simulink model "ControlerModel"  (R2022a)
settings: Solver=VariableStepAuto  StartTime=0.0  StopTime=4  RelTol=1e-3
libraries: simulink_extras x3
settings Model: Creator=Abdullah Syed  LastModifiedBy=Abdullah Syed

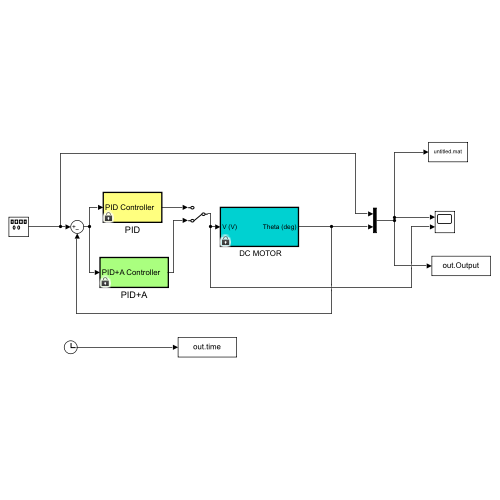
[thumbnail: Simulink's stored preview of the top-level diagram]
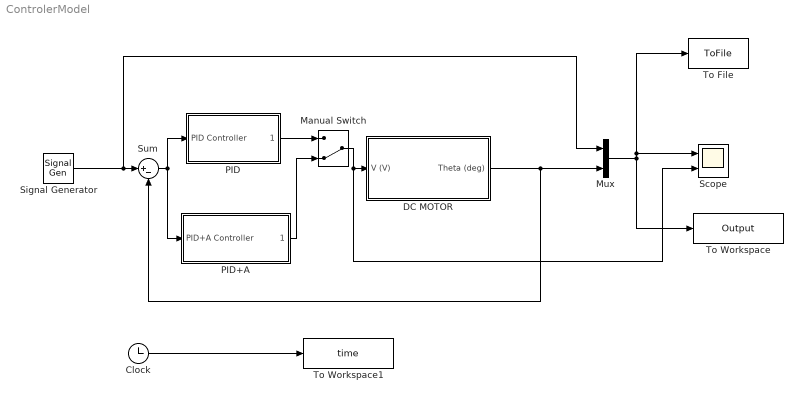
== system ControlerModel ==
  " DC MOTOR" : Subsystem  TreatAsAtomicUnit=on  mask(Single-Tank Nonlinear Model){La=2e-04, Ra=3.5, Jm=3.4700e-07, Bm=1.3319e-07}
      mask prompts: La "Armature Inductance - La (H)"; Ra "Armature Resistance - Ra (ohm)"; Jm "Motor Inertia - Jm (oz.in.sec^2)"; Bm "Motor Viscous Friction - Bm (N.m.sec)"
      mask help: The DC Motor model with saturaton and dead-zone nonlinearities.
      settings: MinAlgLoopOccurrences=on
  Clock : Clock
  Manual Switch : ManualSwitch  CurrentSetting=0
  Mux : Mux  Inputs=2
  PID : Subsystem  TreatAsAtomicUnit=on  mask{Kp=0.52, Ti=5, Td=0}
      mask prompts: Kp "Proportional Gain (Kp)"; Ti "Integral Time Constant (Ti)"; Td "Derivative Time Constant (Td)"
      mask help: This block implements continous PID controller in ideal structure.
      settings: MinAlgLoopOccurrences=on
  PID+A : Subsystem  TreatAsAtomicUnit=on  mask{Kp=0.45, Ti=1.5, Td=0, Kw=7}
      mask prompts: Kp "Proportional Gain (Kp)"; Ti "Integral Time Constant (Ti)"; Td "Derivative Time Constant (Td)"; Kw "Anti-Windup Gain (Kw)"
      mask help: This block implements continous PID controller in ideal structure.
      settings: MinAlgLoopOccurrences=on
  Scope : Scope  NumInputPorts=2
  Signal Generator : SignalGenerator  WaveForm=square  Amplitude=200
  Sum : Sum  Inputs=|+-
  To File : ToFile  SaveFormat=Timeseries
  To Workspace : ToWorkspace  VariableName=Output  SampleTime=-1
  To Workspace1 : ToWorkspace  VariableName=time  SampleTime=-1
  wires:
  Mux/1 -> To File/1, Scope/1, To Workspace/1
  Signal Generator/1 -> Mux/1, Sum/1
  Clock/1 -> To Workspace1/1
  " DC MOTOR"/1(Theta (deg)) -> Mux/2, Sum/2
  Sum/1 -> PID/1(PID Controller), PID+A/1(PID+A Controller)
  Manual Switch/1 -> " DC MOTOR"/1(V (V)), Scope/2
  PID/1("   ") -> Manual Switch/1
  PID+A/1("   ") -> Manual Switch/2

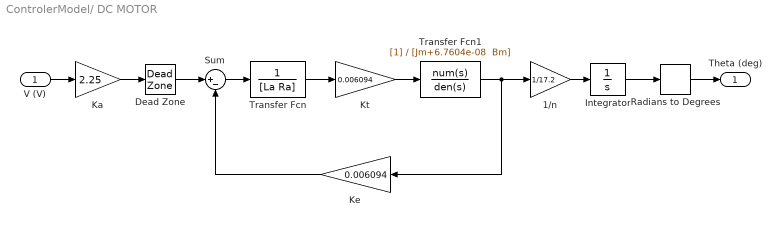
== system ControlerModel/ DC MOTOR ==
  V (V) : Inport
  1/n : Gain  Gain=1/17.2
  Dead Zone : DeadZone  LowerValue=-0.1  UpperValue=0.08  ZeroCross=off
  Integrator : TransferFcn  Denominator=[1 0]
  Ka : Gain  Gain=2.25
  Ke : Gain  Gain=0.006094
  Kt : Gain  Gain=0.006094
  Radians to Degrees : simulink_extras/Transformations/Radians to Degrees
  Sum : Sum  Inputs=|+-
  Transfer Fcn : TransferFcn  Denominator=[La Ra]
  Transfer Fcn1 : TransferFcn  Denominator="[Jm+6.7604e-08  Bm]"
  Theta (deg) : Outport
  wires:
  Sum/1 -> Transfer Fcn/1
  Integrator/1 -> Radians to Degrees/1
  Transfer Fcn/1 -> Kt/1
  Kt/1 -> Transfer Fcn1/1
  Transfer Fcn1/1 -> Ke/1, 1/n/1
  1/n/1 -> Integrator/1
  Ke/1 -> Sum/2
  Dead Zone/1 -> Sum/1
  V (V)/1 -> Ka/1
  Ka/1 -> Dead Zone/1
  Radians to Degrees/1 -> Theta (deg)/1

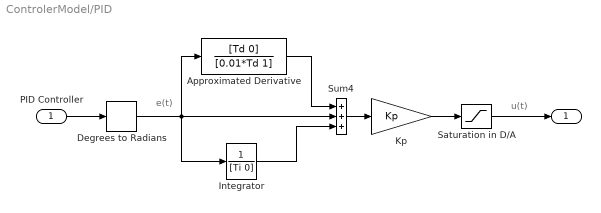
== system ControlerModel/PID ==
  note: e(t)
  note: u(t)
  PID Controller : Inport
  Approximated Derivative : TransferFcn  Numerator=[Td 0]  Denominator=[0.01*Td 1]
  Degrees to Radians : simulink_extras/Transformations/Degrees to Radians
  Integrator : TransferFcn  Denominator=[Ti 0]
  "Kp " : Gain  Gain=Kp
  Saturation in D/A : Saturate  UpperLimit=1.8  LowerLimit=-1.8  ZeroCross=off
  Sum4 : Sum  Inputs=+++
  "   " : Outport
  wires:
  Sum4/1 -> "Kp "/1
  PID Controller/1 -> Degrees to Radians/1
  "Kp "/1 -> Saturation in D/A/1
  Approximated Derivative/1 -> Sum4/1
  Integrator/1 -> Sum4/3
  Saturation in D/A/1 -> "   "/1
  Degrees to Radians/1 -> Approximated Derivative/1, Sum4/2, Integrator/1

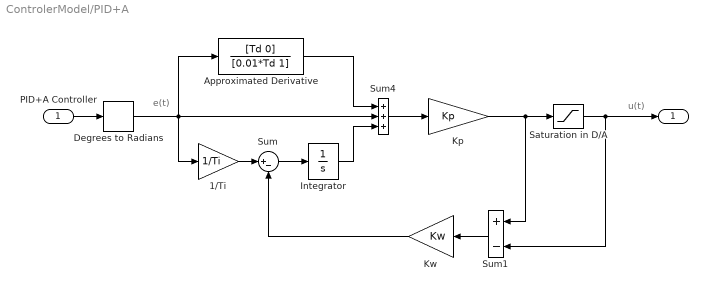
== system ControlerModel/PID+A ==
  note: e(t)
  note: u(t)
  PID+A Controller : Inport
  1/Ti : Gain  Gain=1/Ti
  Approximated Derivative : TransferFcn  Numerator=[Td 0]  Denominator=[0.01*Td 1]
  Degrees to Radians : simulink_extras/Transformations/Degrees to Radians
  Integrator : TransferFcn  Denominator=[1 0]
  "Kp " : Gain  Gain=Kp
  Kw : Gain  Gain=Kw
  Saturation in D/A : Saturate  UpperLimit=1.8  LowerLimit=-1.8  ZeroCross=off
  Sum : Sum  Inputs=|+-
  Sum1 : Sum  Inputs=+-
  Sum4 : Sum  Inputs=+++
  "   " : Outport
  wires:
  Sum4/1 -> "Kp "/1
  PID+A Controller/1 -> Degrees to Radians/1
  "Kp "/1 -> Sum1/1, Saturation in D/A/1
  Approximated Derivative/1 -> Sum4/1
  Saturation in D/A/1 -> Sum1/2, "   "/1
  Sum1/1 -> Kw/1
  Integrator/1 -> Sum4/3
  Sum/1 -> Integrator/1
  1/Ti/1 -> Sum/1
  Kw/1 -> Sum/2
  Degrees to Radians/1 -> 1/Ti/1, Approximated Derivative/1, Sum4/2
